simulink model "SineSetPoint"  (R2016b)
settings: Solver=FixedStepAuto  StartTime=0.0  StopTime=10.0  FixedStep=0.002  RelTol=1e-3  EnableMultiTasking=on
PreLoadFcn:
  | sine_set_point
settings Model: Creator=march  LastModifiedBy=march
settings SolverCC: EnableConcurrentExecution=on
settings DataIOCC: SaveFormat=StructureWithTime
settings OptimizationCC: BlockReduction=off  OptimizeBlockIOStorage=off  BufferReuse=off  GlobalBufferReuse=off  ExpressionFolding=off  LocalBlockOutputs=off
settings HardwareCC: ProdBitPerPointer=32  ProdBitPerSizeT=32  ProdBitPerPtrDiffT=32  ProdLargestAtomicFloat=None  ProdWordSize=32  ProdLongLongMode=on  ProdHWDeviceType=Generic->32-bit x86 compatible
settings RTWCC: SystemTargetFile=slrt.tlc  TemplateMakefile=slrt_default_tmf  Description=Simulink Real-Time  RTWCompilerOptimization=on

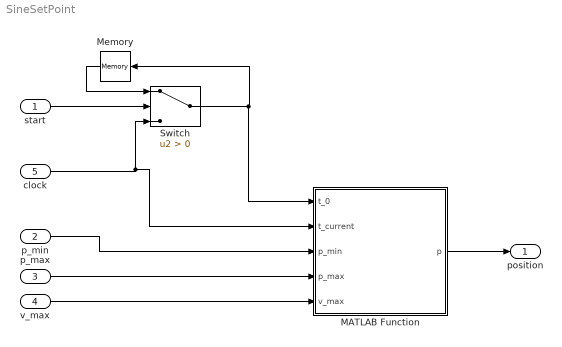
== system SineSetPoint ==
  start : Inport
  p_min : Inport  Port=2
  "p_max " : Inport  Port=3
  v_max : Inport  Port=4
  clock : Inport  Port=5
  MATLAB Function : MATLAB Function  TreatAsAtomicUnit=on
  Memory : Memory
  Switch : Switch  Criteria=u2 > Threshold
  "position " : Outport
  wires:
  Switch/1 -> MATLAB Function/1(t_0), Memory/1
  start/1 -> Switch/2
  clock/1 -> MATLAB Function/2(t_current), Switch/3
  Memory/1 -> Switch/1
  p_min/1 -> MATLAB Function/3(p_min)
  "p_max "/1 -> MATLAB Function/4(p_max)
  v_max/1 -> MATLAB Function/5(v_max)
  MATLAB Function/1(p) -> "position "/1

== matlab function SineSetPoint/MATLAB Function ==
  data: t_0 input; p output; t_current input; p_min input; p_max input; v_max input
function p = sine_set_point(t_0,t_current,p_min,p_max,v_max)
t = t_current-t_0;
ampl_tick = (p_max - p_min)/2; %[ticks]
p_0 = (p_max+p_min)/2;
ampl_rad = ampl_tick/65536*2*pi;%[rad] convert tick to radiants
v_rad = v_max/60*2*pi;%[rad/s] converting RPM to radians per second
f = v_rad / (2*pi*ampl_rad);

p_rad = ampl_rad*sin(t*2*pi*f);
p_tick = p_rad/(2*pi)*65536;

p = p_tick + p_0;
